simulink model "chap3closeLoopN"  (R2020a)
settings: Solver=VariableStepAuto  StartTime=0.0  StopTime=10.0  RelTol=1e-3
libraries: simulink x1, powerlib x1
settings Model: Creator=liuzhenjie  LastModifiedBy=liuzhenjie

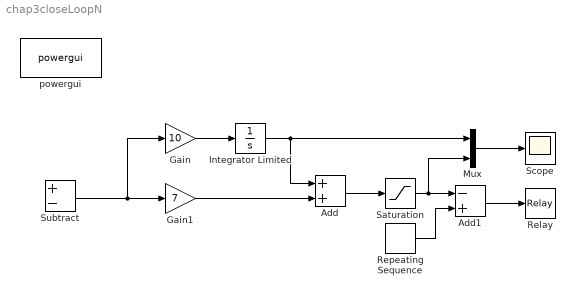
== system chap3closeLoopN ==
  Add : Sum
  Add1 : Sum  Inputs=-+
  Gain : Gain  Gain=10
  Gain1 : Gain  Gain=7
  Integrator Limited : Integrator  LimitOutput=on  UpperSaturationLimit=1  LowerSaturationLimit=0
  Mux : Mux  Inputs=2
  Relay : Relay
  Repeating Sequence : simulink/Sources/Repeating Sequence  rep_seq_t=[0 2]  rep_seq_y=[0 2]
  Saturation : Saturate
  Scope : Scope
  Subtract : Sum  Inputs=+-
  powergui : powerlib/powergui  Priority=1  SimulationMode=Continuous  SampleTime=50e-6  frequency=60  Iterations=50  frequencyindice=60  Pbase=100e6  ErrMax=1e-4  UnitsV=kV  UnitsW=MW  buscounter=0  FunctionMessages=off  echomessages=off  EnableUseOfTLC=off  CurrentSourceSwitches=off  DisableSnubberDevices=off  DisableRonSwitches=off  DisableVfSwitches=off  DisplayEquations=off  AutomaticDiscreteSolvers=off  SolverType=Tustin/Backward Euler (TBE)  Interpol=off  ExternalGateDelay=off  methode=off  Ts=100  x0status=blocks  SPID=on  SwTol=0  HookPort=off  NonlinearTolerance=1e-4  nMaxIteration=100  ContinueOnMaxIteration=off  RestoreLinks=warning  ResistiveCurrentMeasurement=off  Frange=[0:2:500]  Ylog=off  Xlog=on  ShowGrid=off  save=off  variable=ZData  structure=0  ZoomFFT=off  StartTime=0.0  cycles=1  DisplayStyle=1  fundamental=60  FreqAxis=off  MaxFrequency=1000  frequencyindicesteady=1  RmsSteady=1  display=off
  wires:
  Subtract/1 -> Gain/1, Gain1/1
  Gain/1 -> Integrator Limited/1
  Gain1/1 -> Add/2
  Integrator Limited/1 -> Mux/1, Add/1
  Add/1 -> Saturation/1
  Add1/1 -> Relay/1
  Repeating Sequence/1 -> Add1/2
  Mux/1 -> Scope/1
  Saturation/1 -> Mux/2, Add1/1
